simulink model "test_libMdl_Gnss"  (R2018a)
settings: Solver=FixedStepAuto  StartTime=0.0  StopTime=50  RelTol=1e-3
libraries: dspstat3 x6, libMdl_Gnss x1, simulink x1
settings Model: Creator=hwinter  LastModifiedBy=hwinter

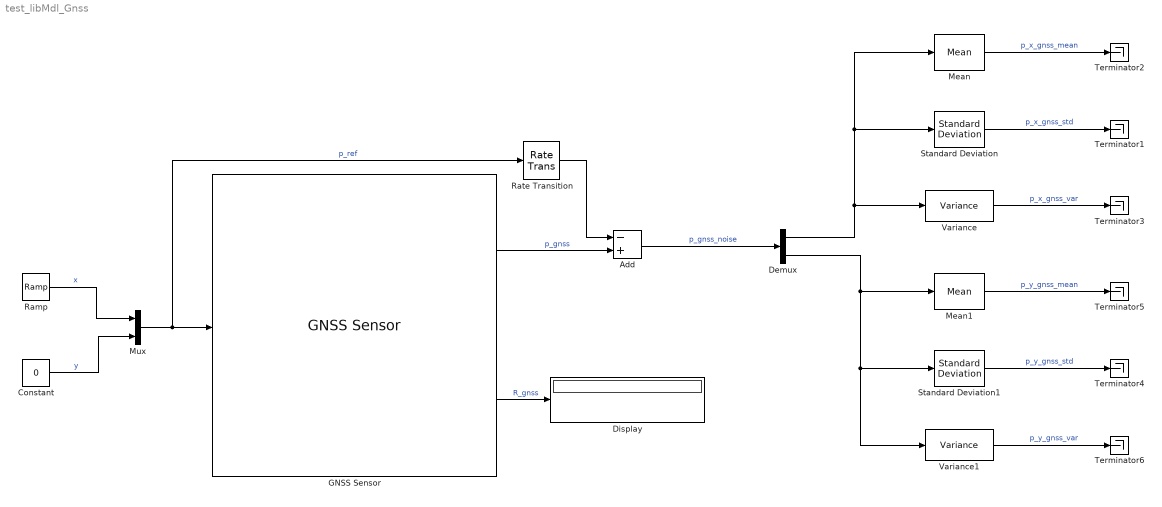
== system test_libMdl_Gnss ==
  Add : Sum  Inputs=-+
  Constant : Constant  Value=0
  Demux : Demux  Outputs=2
  Display : Display
  GNSS Sensor : libMdl_Gnss/GNSS Sensor  mv_T_gnss=0.01  mv_sigma_gnss=[1 1]  mv_z_0_gnss=[0 0]  mv_seed_gnss=654
  Mean : dspstat3/Mean  run=on  InputProcessing=Columns as channels (frame based)  reset_popup=None  directionMode=Each column  dimension=1  roiEnable=off  roiType=Rectangles  roiPortion=Entire ROI  roiOutput=Individual statistics for each ROI  roiFlag=off  roundingMode=Floor  overflowMode=off  outputDataTypeStr=Inherit: Same as accumulator  outputMin=[]  outputMax=[]  outputLastDataTypeStr=Inherit: Same as accumulator
  Mean1 : dspstat3/Mean  run=on  InputProcessing=Columns as channels (frame based)  reset_popup=None  directionMode=Each column  dimension=1  roiEnable=off  roiType=Rectangles  roiPortion=Entire ROI  roiOutput=Individual statistics for each ROI  roiFlag=off  roundingMode=Floor  overflowMode=off  outputDataTypeStr=Inherit: Same as accumulator  outputMin=[]  outputMax=[]  outputLastDataTypeStr=Inherit: Same as accumulator
  Mux : Mux  Inputs=2
  Ramp : simulink/Sources/Ramp  slope=1  start=0  InitialOutput=0
  Rate Transition : RateTransition
  Standard Deviation : dspstat3/Standard Deviation  run=on  directionMode=Each column  dimension=1  InputProcessing=Columns as channels (frame based)  reset_popup=None  roiEnable=off  roiType=Rectangles  roiPortion=Entire ROI  roiOutput=Individual statistics for each ROI  roiFlag=off
      settings: SourceProductName=DSP System Toolbox  SourceProductBaseCode=DS
  Standard Deviation1 : dspstat3/Standard Deviation  run=on  directionMode=Each column  dimension=1  InputProcessing=Columns as channels (frame based)  reset_popup=None  roiEnable=off  roiType=Rectangles  roiPortion=Entire ROI  roiOutput=Individual statistics for each ROI  roiFlag=off
      settings: SourceProductName=DSP System Toolbox  SourceProductBaseCode=DS
  Terminator{1..6} (6 alike) : Terminator
  Variance : dspstat3/Variance  run=on  InputProcessing=Columns as channels (frame based)  reset_popup=None  directionMode=Each column  dimension=1  roiEnable=off  roiType=Rectangles  roiPortion=Entire ROI  roiOutput=Individual statistics for each ROI  roiFlag=off  roundingMode=Floor  overflowMode=off
      settings: SourceProductName=DSP System Toolbox
  Variance1 : dspstat3/Variance  run=on  InputProcessing=Columns as channels (frame based)  reset_popup=None  directionMode=Each column  dimension=1  roiEnable=off  roiType=Rectangles  roiPortion=Entire ROI  roiOutput=Individual statistics for each ROI  roiFlag=off  roundingMode=Floor  overflowMode=off
      settings: SourceProductName=DSP System Toolbox
  wires:
  Constant/1 -> Mux/2  "y"
  Mux/1 -> Rate Transition/1, GNSS Sensor/1  "p_ref"
  Ramp/1 -> Mux/1  "x"
  GNSS Sensor/2 -> Display/1  "R_gnss"
  Mean/1 -> Terminator2/1  "p_x_gnss_mean"
  Standard Deviation/1 -> Terminator1/1  "p_x_gnss_std"
  Variance/1 -> Terminator3/1  "p_x_gnss_var"
  Variance1/1 -> Terminator6/1  "p_y_gnss_var"
  Standard Deviation1/1 -> Terminator4/1  "p_y_gnss_std"
  Mean1/1 -> Terminator5/1  "p_y_gnss_mean"
  Demux/1 -> Mean/1, Standard Deviation/1, Variance/1
  Demux/2 -> Variance1/1, Standard Deviation1/1, Mean1/1
  Add/1 -> Demux/1  "p_gnss_noise"
  GNSS Sensor/1 -> Add/2  "p_gnss"
  Rate Transition/1 -> Add/1
